simulink model "CusakisME4901delay"  (R2013a)
settings: Solver=ode4  StartTime=0.0  StopTime=inf  FixedStep=0.1  RelTol=1e-3
InitFcn:
  | STEPS=14;
  | STEPVEC=[1 1 1 2 2 2 2 3 3 3 4 4 4 4].';
  | TimeStepAct=0.1;
  | f13=3;%second of second and fourth phase
  | f24=4;%second of second and fourth phase
undefined symbols (not defined in the file or in its folder): serial
libraries: instrumentlib x5, simulink x2, aerolibanimutils x1, vrlib x1
settings Model: Creator=Grompone  LastModifiedBy=Grompone

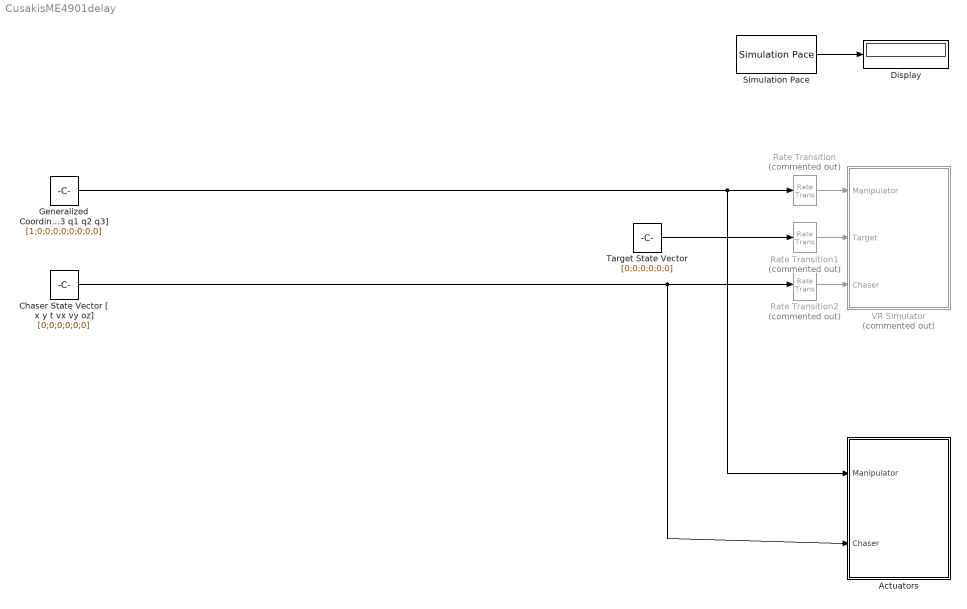
== system CusakisME4901delay ==
  Actuators : Subsystem
  "Chaser State Vector [ x y t vx vy oz] " : Constant  Value=[0;0;0;0;0;0]
  Display : Display
  Generalized Coordinates [qdd1 qdd2 qdd3 qd1 qd2 qd3 q1 q2 q3] : Constant  Value=[1;0;0;0;0;0;0;0;0]
  Rate Transition : RateTransition  Commented=on  OutPortSampleTime=0.2
  Rate Transition1 : RateTransition  Commented=on  OutPortSampleTime=0.2
  Rate Transition2 : RateTransition  Commented=on  OutPortSampleTime=0.2
  Simulation Pace : aerolibanimutils/Simulation Pace  SimulationPace=1  SleepMode=MATLAB Thread  OutputPaceError=on  SampleTime=0.01
      settings: AttributesFormatString=%<SimulationPace> sec/sec
  Target State Vector : Constant  Value=[0;0;0;0;0;0]
  VR Simulator : Subsystem  Commented=on
  wires:
  Rate Transition/1 -> VR Simulator/1(Manipulator)
  Rate Transition1/1 -> VR Simulator/2(Target)
  Rate Transition2/1 -> VR Simulator/3(Chaser)
  Simulation Pace/1 -> Display/1
  "Chaser State Vector [ x y t vx vy oz] "/1 -> Actuators/2(Chaser), Rate Transition2/1
  Target State Vector/1 -> Rate Transition1/1
  Generalized Coordinates [qdd1 qdd2 qdd3 qd1 qd2 qd3 q1 q2 q3]/1 -> Actuators/1(Manipulator), Rate Transition/1

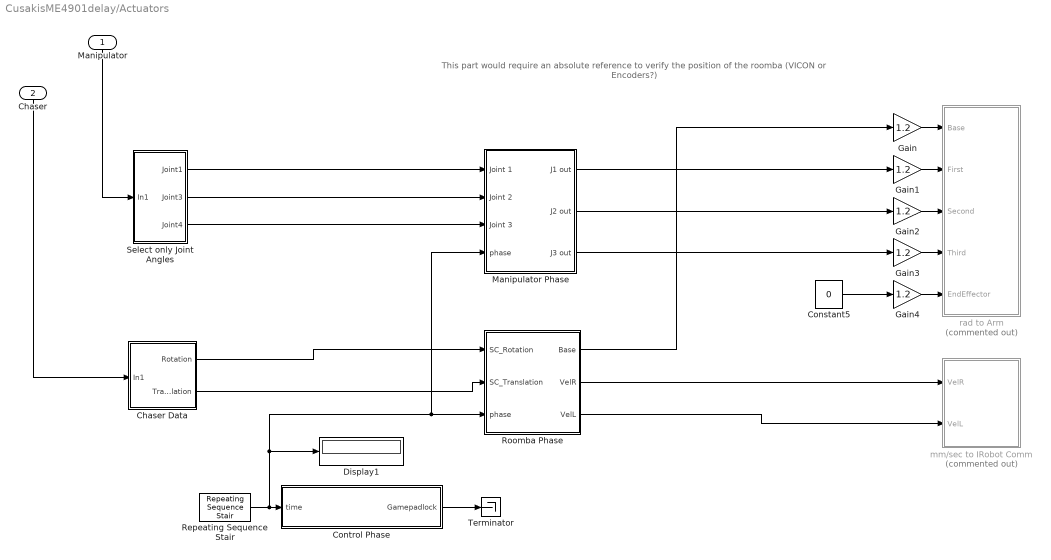
== system CusakisME4901delay/Actuators ==
  note: This part would require an absolute reference to verify the position of the roomba (VICON or Encoders?)
  Manipulator : Inport
  Chaser : Inport  Port=2
  Chaser Data : Subsystem
  Constant5 : Constant  Value=0
  Control Phase : MATLAB Function  TreatAsAtomicUnit=on
  Display1 : Display
  Gain{,1..4} (5 alike) : Gain  Gain=1.2
  Manipulator Phase : Subsystem
  Repeating Sequence Stair : simulink/Sources/Repeating Sequence Stair  OutValues=STEPVEC  tsamp=1  OutMin=[]  OutMax=[]  OutDataTypeStr=double  OutputDataTypeScalingMode=double  OutDataType=fixdt(0,8)  ConRadixGroup=Best Precision: Vector-wise  OutScaling=2^-12
  Roomba Phase : Subsystem
  Select only Joint Angles : Subsystem
  Terminator : Terminator
  mm/sec to IRobot Comm : Subsystem  Commented=on
  rad to Arm : Subsystem  Commented=on
  wires:
  Chaser/1 -> Chaser Data/1(In1)
  Manipulator/1 -> Select only Joint Angles/1(In1)
  Constant5/1 -> Gain4/1
  Chaser Data/2(Translation) -> Roomba Phase/2(SC_Translation)
  Select only Joint Angles/3(Joint4) -> Manipulator Phase/3(Joint 3)
  Select only Joint Angles/2(Joint3) -> Manipulator Phase/2(Joint 2)
  Select only Joint Angles/1(Joint1) -> Manipulator Phase/1(Joint 1)
  Gain/1 -> rad to Arm/1(Base)
  Gain1/1 -> rad to Arm/2(First)
  Gain2/1 -> rad to Arm/3(Second)
  Gain3/1 -> rad to Arm/4(Third)
  Gain4/1 -> rad to Arm/5(EndEffector)
  Chaser Data/1(Rotation) -> Roomba Phase/1(SC_Rotation)
  Manipulator Phase/1(J1 out) -> Gain1/1
  Manipulator Phase/2(J2 out) -> Gain2/1
  Manipulator Phase/3(J3 out) -> Gain3/1
  Repeating Sequence Stair/1 -> Manipulator Phase/4(phase), Roomba Phase/3(phase), Display1/1, Control Phase/1(time)
  Control Phase/1(Gamepadlock) -> Terminator/1
  Roomba Phase/2(VelR) -> mm/sec to IRobot Comm/1(VelR)
  Roomba Phase/3(VelL) -> mm/sec to IRobot Comm/2(VelL)
  Roomba Phase/1(Base) -> Gain/1

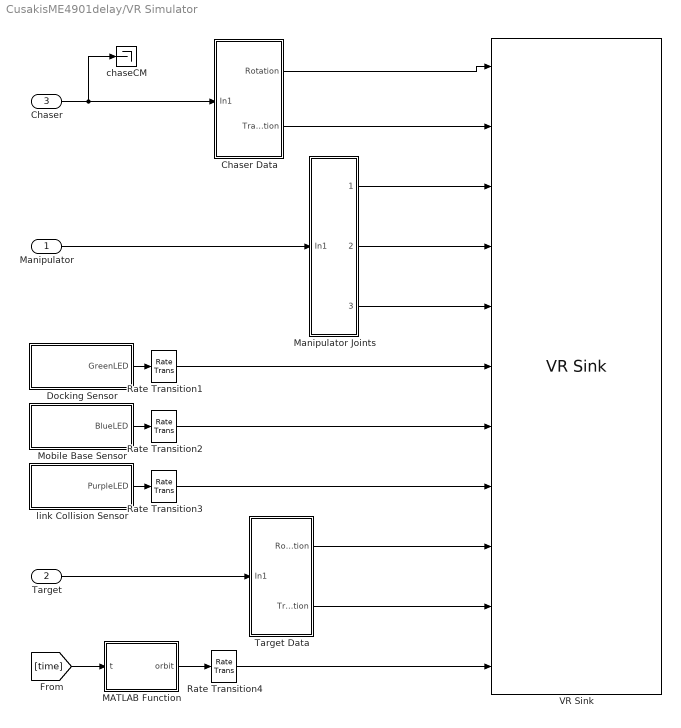
== system CusakisME4901delay/VR Simulator ==
  Manipulator : Inport
  Target : Inport  Port=2
  Chaser : Inport  Port=3
  Chaser Data : Subsystem
  Docking Sensor : Subsystem
  MATLAB Function : MATLAB Function  TreatAsAtomicUnit=on
  Manipulator Joints : Subsystem
  Mobile Base Sensor : Subsystem
  Rate Transition{1..4} (4 alike) : RateTransition  OutPortSampleTime=0.2
  Target Data : Subsystem
  VR Sink : vrlib/VR Sink  InstantiateOnLoad=on  SampleTime=0.2  ViewEnable=on  RemoteChange=off  RemoteView=off  FieldsWritten=CHASER.rotation.4.1.1.double#CHASER.translation.3.1.1.double#Joint1.rotation.4.1.1.double#Joint2.rotation.4.1.1.double#Joint3.rotation.4.1.1.double#we.diffuseColor.3.1.1.double#g.diffuseColor.3.1.1.double#Cl.diffuseColor.3.1.1.double#TARGET.rotation.4.1.1.double#TARGET.translation.3.1.1.double#Otherview.translation.3.1.1.double  WorldFileName=final1b.wrl  AutoView=off  VideoDimensions=[]  AllowVariableSize=off
  chaseCM : Terminator
  link Collision Sensor : Subsystem
  wires:
  Manipulator/1 -> Manipulator Joints/1(In1)
  Target/1 -> Target Data/1(In1)
  [time] -> MATLAB Function/1(t)
  Chaser/1 -> chaseCM/1, Chaser Data/1(In1)
  Chaser Data/1(Rotation) -> VR Sink/1
  Chaser Data/2(Translation) -> VR Sink/2
  Manipulator Joints/1(Joint1) -> VR Sink/3
  Manipulator Joints/3(Joint4) -> VR Sink/5
  Target Data/1(Rotation) -> VR Sink/9
  Target Data/2(Translation) -> VR Sink/10
  MATLAB Function/1(orbit) -> Rate Transition4/1
  link Collision Sensor/1(PurpleLED) -> Rate Transition3/1
  Docking Sensor/1(GreenLED) -> Rate Transition1/1
  Mobile Base Sensor/1(BlueLED) -> Rate Transition2/1
  Manipulator Joints/2(Joint3) -> VR Sink/4
  Rate Transition1/1 -> VR Sink/6
  Rate Transition2/1 -> VR Sink/7
  Rate Transition3/1 -> VR Sink/8
  Rate Transition4/1 -> VR Sink/11

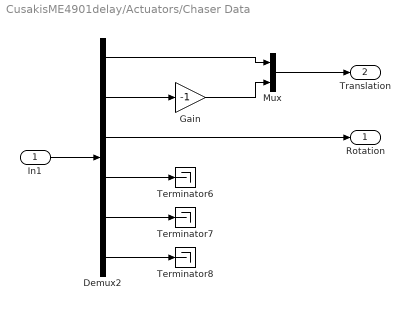
== system CusakisME4901delay/Actuators/Chaser Data ==
  In1 : Inport
  Demux2 : Demux  Outputs=6
  Gain : Gain  Gain=-1
  Mux : Mux  Inputs=2
  Terminator6 : Terminator
  Terminator7 : Terminator
  Terminator8 : Terminator
  Rotation : Outport
  Translation : Outport  Port=2
  wires:
  In1/1 -> Demux2/1
  Demux2/5 -> Terminator7/1
  Demux2/4 -> Terminator6/1
  Demux2/2 -> Gain/1
  Mux/1 -> Translation/1
  Demux2/1 -> Mux/1
  Gain/1 -> Mux/2
  Demux2/3 -> Rotation/1
  Demux2/6 -> Terminator8/1

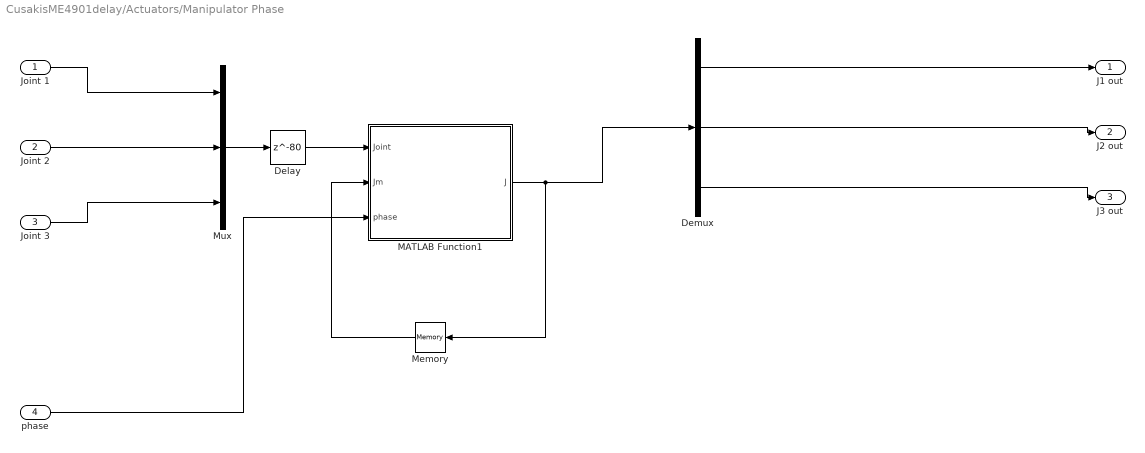
== system CusakisME4901delay/Actuators/Manipulator Phase ==
  Joint 1 : Inport
  Joint 2 : Inport  Port=2
  Joint 3 : Inport  Port=3
  phase : Inport  Port=4
  Delay : Delay  DelayLength=80  InitialCondition=0  SampleTime=0.1
  Demux : Demux  Outputs=3
  MATLAB Function1 : MATLAB Function  TreatAsAtomicUnit=on
  Memory : Memory  X0=[0;0;0]
  Mux : Mux  Inputs=3
  J1 out : Outport
  J2 out : Outport  Port=2
  J3 out : Outport  Port=3
  wires:
  Joint 1/1 -> Mux/1
  Joint 2/1 -> Mux/2
  Joint 3/1 -> Mux/3
  Mux/1 -> Delay/1
  Demux/1 -> J1 out/1
  Demux/2 -> J2 out/1
  Demux/3 -> J3 out/1
  MATLAB Function1/1(J) -> Memory/1, Demux/1
  Memory/1 -> MATLAB Function1/2(Jm)
  phase/1 -> MATLAB Function1/3(phase)
  Delay/1 -> MATLAB Function1/1(Joint)

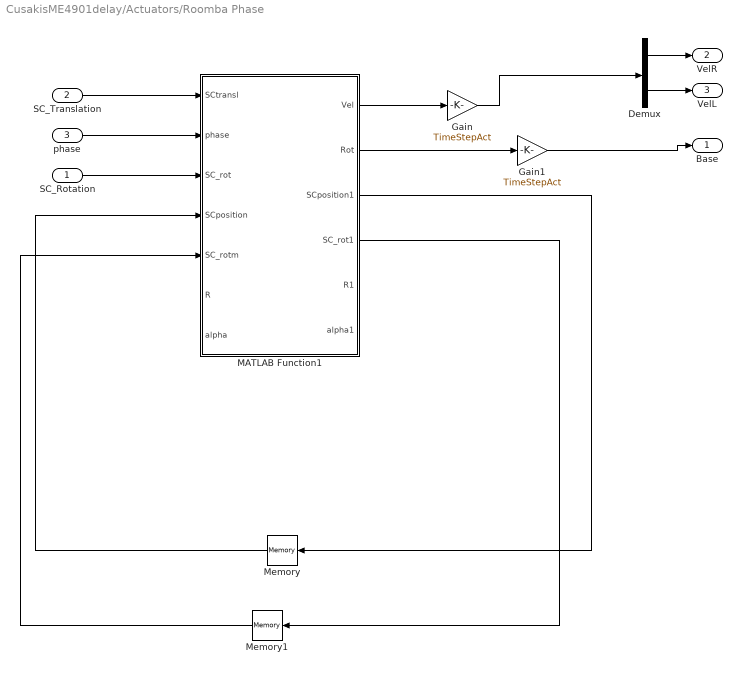
== system CusakisME4901delay/Actuators/Roomba Phase ==
  SC_Rotation : Inport
  SC_Translation : Inport  Port=2
  phase : Inport  Port=3
  Demux : Demux  Outputs=2
  Gain : Gain  Gain=TimeStepAct
  Gain1 : Gain  Gain=TimeStepAct
  MATLAB Function1 : MATLAB Function  TreatAsAtomicUnit=on
  Memory : Memory  X0=[0;0;0]
  Memory1 : Memory
  Base : Outport
  VelR : Outport  Port=2
  VelL : Outport  Port=3
  wires:
  Demux/1 -> VelR/1
  Demux/2 -> VelL/1
  SC_Rotation/1 -> MATLAB Function1/3(SC_rot)
  phase/1 -> MATLAB Function1/2(phase)
  SC_Translation/1 -> MATLAB Function1/1(SCtransl)
  Memory/1 -> MATLAB Function1/4(SCposition)
  Memory1/1 -> MATLAB Function1/5(SC_rotm)
  MATLAB Function1/1(Vel) -> Gain/1
  MATLAB Function1/2(Rot) -> Gain1/1
  MATLAB Function1/3(SCposition1) -> Memory/1
  MATLAB Function1/4(SC_rot1) -> Memory1/1
  Gain/1 -> Demux/1
  Gain1/1 -> Base/1

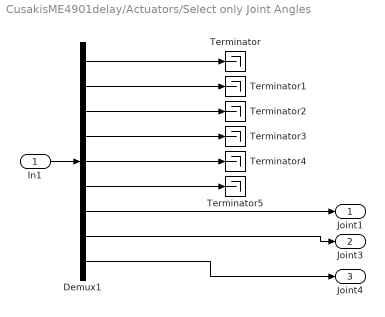
== system CusakisME4901delay/Actuators/Select only Joint Angles ==
  In1 : Inport
  Demux1 : Demux  Outputs=9
  Terminator{,1..5} (6 alike) : Terminator
  Joint1 : Outport
  Joint3 : Outport  Port=2
  Joint4 : Outport  Port=3
  wires:
  Demux1/9 -> Joint4/1
  Demux1/8 -> Joint3/1
  Demux1/7 -> Joint1/1
  Demux1/6 -> Terminator5/1
  Demux1/5 -> Terminator4/1
  Demux1/4 -> Terminator3/1
  Demux1/3 -> Terminator2/1
  Demux1/2 -> Terminator1/1
  Demux1/1 -> Terminator/1
  In1/1 -> Demux1/1

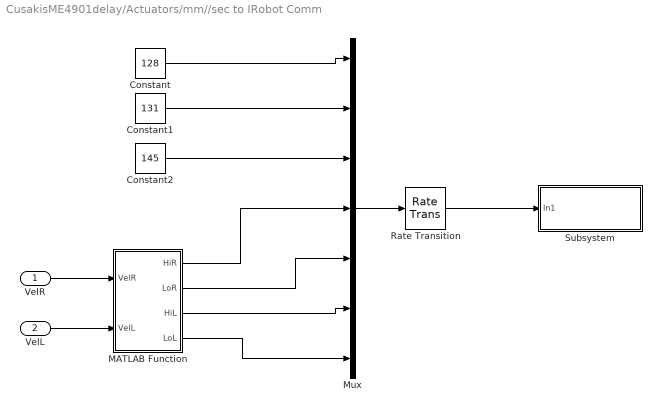
== system CusakisME4901delay/Actuators/mm//sec to IRobot Comm ==
  VelR : Inport
  VelL : Inport  Port=2
  Constant : Constant  Value=128  OutDataTypeStr=uint8
  Constant1 : Constant  Value=131  OutDataTypeStr=uint8
  Constant2 : Constant  Value=145  OutDataTypeStr=uint8
  MATLAB Function : MATLAB Function  TreatAsAtomicUnit=on
  Mux : Mux  Inputs=7
  Rate Transition : RateTransition  OutPortSampleTime=1
  Subsystem : Subsystem
  wires:
  MATLAB Function/1(HiR) -> Mux/4
  MATLAB Function/2(LoR) -> Mux/5
  MATLAB Function/3(HiL) -> Mux/6
  MATLAB Function/4(LoL) -> Mux/7
  VelR/1 -> MATLAB Function/1(VelR)
  VelL/1 -> MATLAB Function/2(VelL)
  Constant/1 -> Mux/1
  Constant1/1 -> Mux/2
  Constant2/1 -> Mux/3
  Mux/1 -> Rate Transition/1
  Rate Transition/1 -> Subsystem/1(In1)

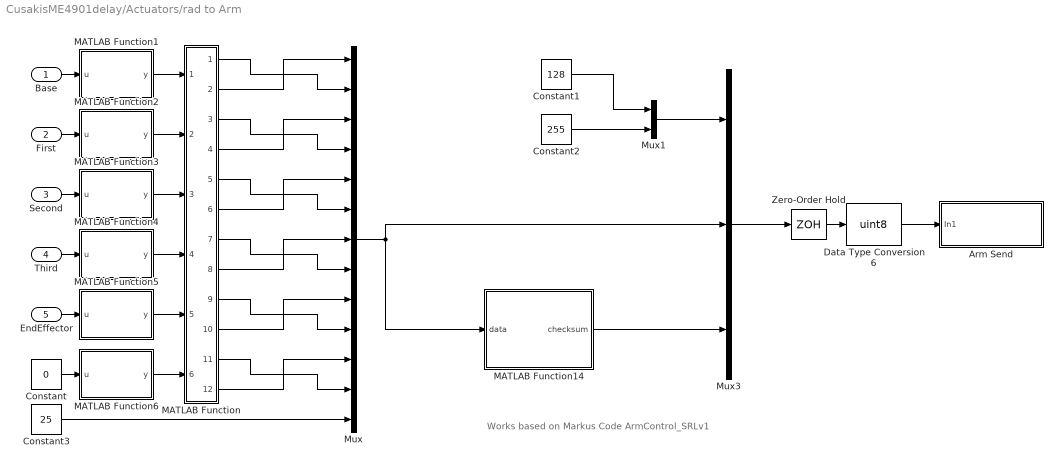
== system CusakisME4901delay/Actuators/rad to Arm ==
  note: Works based on Markus Code ArmControl_SRLv1
  Base : Inport
  First : Inport  Port=2
  Second : Inport  Port=3
  Third : Inport  Port=4
  EndEffector : Inport  Port=5
  Arm Send : Subsystem
  Constant : Constant  Value=0  OutDataTypeStr=uint8
  Constant1 : Constant  Value=128  OutDataTypeStr=uint8
  Constant2 : Constant  Value=255  OutDataTypeStr=uint8
  Constant3 : Constant  Value=25  OutDataTypeStr=uint8
  Data Type Conversion6 : DataTypeConversion  OutDataTypeStr=uint8
  MATLAB Function : MATLAB Function  TreatAsAtomicUnit=on
  MATLAB Function1 : MATLAB Function  TreatAsAtomicUnit=on
  MATLAB Function14 : MATLAB Function  TreatAsAtomicUnit=on
  MATLAB Function2 : MATLAB Function  TreatAsAtomicUnit=on
  MATLAB Function3 : MATLAB Function  TreatAsAtomicUnit=on
  MATLAB Function4 : MATLAB Function  TreatAsAtomicUnit=on
  MATLAB Function5 : MATLAB Function  TreatAsAtomicUnit=on
  MATLAB Function6 : MATLAB Function  TreatAsAtomicUnit=on
  Mux : Mux  Inputs=13
  Mux1 : Mux  Inputs=2
  Mux3 : Mux  Inputs=3
  Zero-Order Hold : ZeroOrderHold  SampleTime=0.01
  wires:
  EndEffector/1 -> MATLAB Function5/1(u)
  First/1 -> MATLAB Function2/1(u)
  Second/1 -> MATLAB Function3/1(u)
  Third/1 -> MATLAB Function4/1(u)
  Base/1 -> MATLAB Function1/1(u)
  Constant/1 -> MATLAB Function6/1(u)
  Constant1/1 -> Mux1/1
  Constant2/1 -> Mux1/2
  Constant3/1 -> Mux/13
  MATLAB Function14/1(checksum) -> Mux3/3
  Mux/1 -> Mux3/2, MATLAB Function14/1(data)
  Mux1/1 -> Mux3/1
  Data Type Conversion6/1 -> Arm Send/1(In1)
  MATLAB Function/2(LoBase) -> Mux/1
  MATLAB Function/4(LoM1) -> Mux/3
  MATLAB Function/6(LoM2) -> Mux/5
  MATLAB Function/8(LoM3) -> Mux/7
  MATLAB Function/10(LoEnd) -> Mux/9
  MATLAB Function/12(LoO) -> Mux/11
  MATLAB Function/1(HiBase) -> Mux/2
  MATLAB Function/3(HiM1) -> Mux/4
  MATLAB Function/5(HiM2) -> Mux/6
  MATLAB Function/7(HiM3) -> Mux/8
  MATLAB Function/9(HiEnd) -> Mux/10
  MATLAB Function/11(HiO) -> Mux/12
  MATLAB Function1/1(y) -> MATLAB Function/1(Base)
  MATLAB Function2/1(y) -> MATLAB Function/2(M1)
  MATLAB Function3/1(y) -> MATLAB Function/3(M2)
  MATLAB Function4/1(y) -> MATLAB Function/4(M3)
  MATLAB Function5/1(y) -> MATLAB Function/5(End)
  MATLAB Function6/1(y) -> MATLAB Function/6(other)
  Mux3/1 -> Zero-Order Hold/1
  Zero-Order Hold/1 -> Data Type Conversion6/1

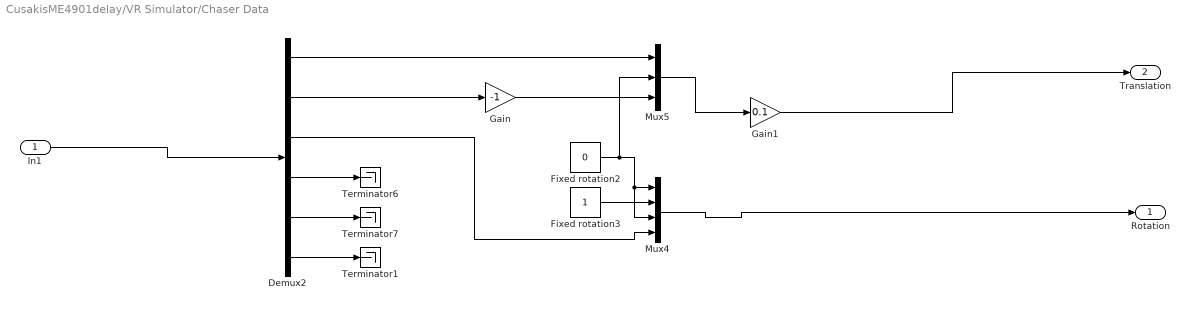
== system CusakisME4901delay/VR Simulator/Chaser Data ==
  In1 : Inport
  Demux2 : Demux  Outputs=6
  Fixed rotation2 : Constant  Value=0
  Fixed rotation3 : Constant
  Gain : Gain  Gain=-1
  Gain1 : Gain  Gain=0.1
  Mux4 : Mux
  Mux5 : Mux  Inputs=3
  Terminator1 : Terminator
  Terminator6 : Terminator
  Terminator7 : Terminator
  Rotation : Outport
  Translation : Outport  Port=2
  wires:
  In1/1 -> Demux2/1
  Mux5/1 -> Gain1/1
  Demux2/5 -> Terminator7/1
  Demux2/4 -> Terminator6/1
  Demux2/2 -> Gain/1
  Fixed rotation2/1 -> Mux4/1, Mux4/3, Mux5/2
  Fixed rotation3/1 -> Mux4/2
  Demux2/3 -> Mux4/4
  Gain1/1 -> Translation/1
  Mux4/1 -> Rotation/1
  Demux2/1 -> Mux5/1
  Gain/1 -> Mux5/3
  Demux2/6 -> Terminator1/1

== system CusakisME4901delay/VR Simulator/Docking Sensor ==
  Fixed translation3 : Constant  Value=[0 0 0]
  Green : Constant  Value=[0.2 1 0.2]
  Rate Transition : RateTransition
  Red : Constant  Value=[1 0 0]
  Repeating Sequence Stair : simulink/Sources/Repeating Sequence Stair  OutValues=[0 1].'  tsamp=0.5  OutMin=[]  OutMax=[]  OutDataTypeStr=double  OutputDataTypeScalingMode=double  OutDataType=fixdt(0,8)  ConRadixGroup=Best Precision: Vector-wise  OutScaling=2^-12
  Switch : Switch  Criteria=u2 ~= 0
  Switch1 : Switch  Criteria=u2 ~= 0
  GreenLED : Outport
  wires:
  [docking] -> Switch/2
  Fixed translation3/1 -> Switch1/3
  Repeating Sequence Stair/1 -> Rate Transition/1
  Green/1 -> Switch/1
  Red/1 -> Switch1/1
  Switch1/1 -> Switch/3
  Rate Transition/1 -> Switch1/2
  Switch/1 -> GreenLED/1

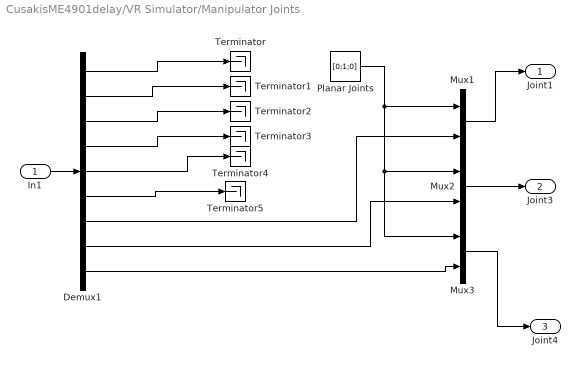
== system CusakisME4901delay/VR Simulator/Manipulator Joints ==
  In1 : Inport
  Demux1 : Demux  Outputs=9
  Mux1 : Mux  Inputs=2
  Mux2 : Mux  Inputs=2
  Mux3 : Mux  Inputs=2
  Planar Joints : Constant  Value=[0;1;0]
  Terminator{,1..5} (6 alike) : Terminator
  Joint1 : Outport
  Joint3 : Outport  Port=2
  Joint4 : Outport  Port=3
  wires:
  In1/1 -> Demux1/1
  Demux1/8 -> Mux2/2
  Demux1/9 -> Mux3/2
  Demux1/7 -> Mux1/2
  Demux1/1 -> Terminator/1
  Demux1/2 -> Terminator1/1
  Demux1/3 -> Terminator2/1
  Demux1/4 -> Terminator3/1
  Demux1/5 -> Terminator4/1
  Demux1/6 -> Terminator5/1
  Planar Joints/1 -> Mux3/1, Mux2/1, Mux1/1
  Mux1/1 -> Joint1/1
  Mux2/1 -> Joint3/1
  Mux3/1 -> Joint4/1

== system CusakisME4901delay/VR Simulator/Mobile Base Sensor ==
  Green : Constant  Value=[0 0 0]
  Green1 : Constant  Value=[0 0 1]
  Switch : Switch  Criteria=u2 ~= 0
  BlueLED : Outport
  wires:
  Switch/1 -> BlueLED/1
  Green/1 -> Switch/1
  [mobilebase] -> Switch/2
  Green1/1 -> Switch/3

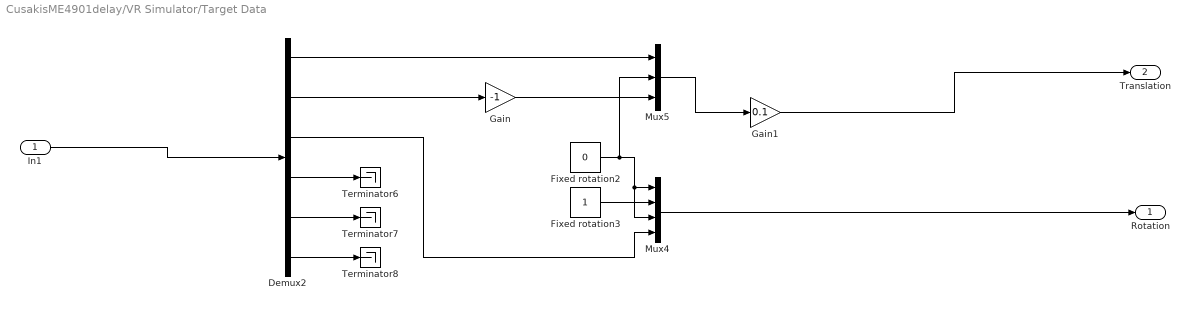
== system CusakisME4901delay/VR Simulator/Target Data ==
  In1 : Inport
  Demux2 : Demux  Outputs=6
  Fixed rotation2 : Constant  Value=0
  Fixed rotation3 : Constant
  Gain : Gain  Gain=-1
  Gain1 : Gain  Gain=0.1
  Mux4 : Mux
  Mux5 : Mux  Inputs=3
  Terminator6 : Terminator
  Terminator7 : Terminator
  Terminator8 : Terminator
  Rotation : Outport
  Translation : Outport  Port=2
  wires:
  Fixed rotation3/1 -> Mux4/2
  Fixed rotation2/1 -> Mux5/2, Mux4/3, Mux4/1
  Demux2/1 -> Mux5/1
  Demux2/2 -> Gain/1
  Demux2/3 -> Mux4/4
  Demux2/4 -> Terminator6/1
  Demux2/5 -> Terminator7/1
  Demux2/6 -> Terminator8/1
  Gain/1 -> Mux5/3
  Mux5/1 -> Gain1/1
  Gain1/1 -> Translation/1
  Mux4/1 -> Rotation/1
  In1/1 -> Demux2/1

== system CusakisME4901delay/VR Simulator/link Collision Sensor ==
  Black : Constant  Value=[0 0 0]
  Purple : Constant  Value=[1 0 1]
  Switch : Switch  Criteria=u2 ~= 0
  PurpleLED : Outport
  wires:
  Black/1 -> Switch/3
  [linkcoll] -> Switch/2
  Purple/1 -> Switch/1
  Switch/1 -> PurpleLED/1

== system CusakisME4901delay/Actuators/mm//sec to IRobot Comm/Subsystem ==
  In1 : Inport
  Serial Configuration : instrumentlib/Serial Configuration  Priority=-200000  ComPortMenu=<Please select a port...>  ComPort=COM4  ObjConstructor=serial('COM4');  BaudRate=57600  DataBits=8  Parity=none  StopBits=1  FlowControl=none  Timeout=10  ByteOrder=LittleEndian
  Serial Send : instrumentlib/Serial Send  ComPortMenu=<Please select a port...>  ComPort=COM4  ObjConstructor=serial('COM4');  Terminator=<none>  EnableBlockingMode=off
  wires:
  In1/1 -> Serial Send/1

== system CusakisME4901delay/Actuators/rad to Arm/Arm Send ==
  In1 : Inport
  Display2 : Display
  Display3 : Display
  Rate Transition : RateTransition  OutPortSampleTime=0.1
  Serial Configuration : instrumentlib/Serial Configuration  Priority=-200000  ComPortMenu=<Please select a port...>  ComPort=COM5  ObjConstructor=serial('COM5');  BaudRate=57600  DataBits=8  Parity=none  StopBits=1  FlowControl=none  Timeout=10  ByteOrder=LittleEndian
  Serial Receive : instrumentlib/Serial Receive  ComPortMenu=<Please select a port...>  ComPort=COM5  ObjConstructor=serial('COM5');  Terminator=<none>  DataSize="[1  16]"  DataType=uint8  EnableBlockingMode=off  ActionDataUnavailable=Output last received value  CustomValue=0  SampleTime=0.1
  Serial Send : instrumentlib/Serial Send  ComPortMenu=<Please select a port...>  ComPort=COM5  ObjConstructor=serial('COM5');  Terminator=<none>  EnableBlockingMode=off
  wires:
  In1/1 -> Rate Transition/1
  Rate Transition/1 -> Serial Send/1
  Serial Receive/1 -> Display2/1
  Serial Receive/2 -> Display3/1

== matlab function CusakisME4901delay/Actuators/Roomba Phase/MATLAB Function1 ==
  data: SCtransl input; phase input; SC_rot input; SCposition input; Vel output; SC_rotm input; R input; alpha input; Rot output; f13 parameter; f24 parameter; SCposition1 output; SC_rot1 output; R1 output; alpha1 output
function [Vel,Rot,SCposition1,SC_rot1,R1,alpha1]  = fcn(SCtransl,phase,SC_rot,SCposition,SC_rotm,R,alpha,f13,f24)
%#codegen

%Inputs
r=0.13; %radius of roomba's wheels
%SCtranslation [ X; Y; Theta; Vx; Vy; Omega ]

%SCposition [X; Y; Theta]

if phase==1 %CONTROL PHASE Operator is giving the inputs and the time history is being computed
    SCposition1=SCposition;
    SC_rot1=SC_rot;
    
    Vel=[0;0];
    Rot=SC_rotm;

elseif phase==2 %ADAPTATION PHASE The base adapts it's attitude in order to be ready to maneuver and the velocities are 0
    SCposition1=SCposition;
    SC_rot1=SC_rot;
    
    Xf=SCposition;
    Xi=SCtransl;
    DeltaSC=[Xf(1)-Xi(1);Xf(2)-Xi(2);Xf(3)-Xi(3)];
    
    R=sqrt(DelataSC(1)^2+DelataSC(2)^2); %distance to maneuvered
    
    alpha=atan2(DeltaSC(2),DeltaSC(1));  %angle to be maneuvered
    
    if alpha>0 && alpha <1.57
        Sl=alpha*(-r);
        Sr=alpha*(r);
    elseif alpha>1.57 && alpha <3.14
        Sl=alpha*(-r);
        Sr=alpha*(r);
    elseif alpha<0 && alpha >-1.57
        Sl=-alpha*(r);
        Sr=-alpha*(-r);
    elseif alpha<-1.57 && alpha >-3.14
        Sl=-alpha*(r);
        Sr=-alpha*(-r);
    end
    
    %this part should be integrated....in steps to regulate velocity!!
    Vel=[Sr/f24;Sl/f24]; %Provides only the angle maneuver
    Rot=-alpha/f24; %the First Link has to compensate this adaptation
     
elseif phase==3 %SIMULATION PHASE Manipulator and base maneuver according to time history
    SCposition1=SCposition;
    SC_rot1=SC_rot;
    
    %Simulates translation of the spacecraft time histories
    Vel=[R/f13;R/f13];
    Rot=SC_rot; %simulates rotations of the spacecraft time histories
    
else %RESET PHASE, Cancels angle between base and Roomba
    SCposition1=SCtransl;
    SC_rot1=SC_rotm;
    
    Rot=SC_rot+Rot; %simulates rotations of the spacecraft time histories
    Vel=[R/f13;R/f13];
    
end

== matlab function CusakisME4901delay/Actuators/Control Phase ==
  data: time input; Gamepadlock output
function Gamepadlock = fcn(time)
%#codegen



if time==1 
    
Gamepadlock=1; 

else
    
Gamepadlock=0;  %Locks the gamepad when the user cannot send data.  

end


%What I Want from this code


% if time<3*n
%     
% Joypad inputs the velocities and the model calculates the generalized
% coordinates and spacecraft position
%
%
% if time>3*n && time<8*n
%
% The model stops computation saves the time history of the gen coordinates
% The Cusakis rotates towards the direction it will have to move
%
%
% if time>8*n && time<11*n
%
% Cusakis moves twoards the new center position and the manipulator uses
% the time history 
%
%

== matlab function CusakisME4901delay/Actuators/Manipulator Phase/MATLAB Function1 ==
  data: Joint input; Jm input; phase input; J output
function J   = fcn(Joint,Jm,phase)
%#codegen

%freeses the manipulator in phase 1 2 and 4


if phase==3 
      J=Joint;
else
    J=Jm;
end

== matlab function CusakisME4901delay/VR Simulator/MATLAB Function ==
  data: t input; orbit output
function orbit = fcn(t)
%#codegen



w=0.01;

x=cos(w*t);

z=sin(w*t);

y=0;

%orbit = [x;y;z];

orbit = [0;0;0];

== matlab function CusakisME4901delay/Actuators/rad to Arm/MATLAB Function1 ==
  data: u input; y output
function y = fcn(u)
%#codegen
udeg=u*180/pi;

%degrees to arduino angles..(avoids negative numbers)
y = (udeg+180)*10;

== matlab function CusakisME4901delay/Actuators/rad to Arm/MATLAB Function2 ==
  data: u input; y output
function y = fcn(u)
%#codegen
udeg=u*180/pi;

%degrees to arduino angles..(avoids negative numbers)
y = (udeg+180)*10;

== matlab function CusakisME4901delay/Actuators/rad to Arm/MATLAB Function3 ==
  data: u input; y output
function y = fcn(u)
%#codegen
udeg=u*180/pi;

%degrees to arduino angles..(avoids negative numbers)
y = (udeg+180)*10;

== matlab function CusakisME4901delay/Actuators/rad to Arm/MATLAB Function4 ==
  data: u input; y output
function y = fcn(u)
%#codegen
udeg=u*180/pi;

%degrees to arduino angles..(avoids negative numbers)
y = (udeg+180)*10;

== matlab function CusakisME4901delay/Actuators/rad to Arm/MATLAB Function5 ==
  data: u input; y output
function y = fcn(u)
%#codegen
udeg=u*180/pi;

%degrees to arduino angles..(avoids negative numbers)
y = (udeg+180)*10;

== matlab function CusakisME4901delay/Actuators/rad to Arm/MATLAB Function ==
  data: Base input; HiBase output; M1 input; LoBase output; HiM1 output; LoM1 output; M2 input; M3 input; End input; HiM2 output; LoM2 output; HiM3 output; LoM3 output; HiEnd output; LoEnd output; other input; HiO output; LoO output
function [HiBase,LoBase,HiM1,LoM1,HiM2,LoM2,HiM3,LoM3,HiEnd,LoEnd,HiO,LoO] = fcn(Base,M1,M2,M3,End,other)
%#codegen


BaseV=typecast(int16(Base),'uint8');
M1V=typecast(int16(M1),'uint8');
M2V=typecast(int16(M2),'uint8');
M3V=typecast(int16(M3),'uint8');
EndV=typecast(int16(End),'uint8');
OtherV=typecast(int16(other),'uint8');


HiBase=BaseV(2);
LoBase=BaseV(1);
HiM1=M1V(2);
LoM1=M1V(1);
HiM2=M2V(2);
LoM2=M2V(1);
HiM3=M3V(2);
LoM3=M3V(1);
HiEnd=EndV(2);
LoEnd=EndV(1);
HiO=OtherV(2);
LoO=OtherV(1);

== matlab function CusakisME4901delay/Actuators/rad to Arm/MATLAB Function14 ==
  data: data input; checksum output
function checksum = Checksum(data)
% Calculates checksum of command signal

data = int16(data);
tempsum = sum(data);
temp = 255 - mod(tempsum,256);

checksum = uint8(temp);

== matlab function CusakisME4901delay/Actuators/rad to Arm/MATLAB Function6 ==
  data: u input; y output
function y = fcn(u)
%#codegen
udeg=u*180/pi;

%degrees to arduino angles..(avoids negative numbers)
y = (udeg+180)*10;

== matlab function CusakisME4901delay/Actuators/mm//sec to IRobot Comm/MATLAB Function ==
  data: VelR input; HiR output; VelL input; LoR output; HiL output; LoL output
function [HiR,LoR,HiL,LoL] = fcn(VelR,VelL)
%#codegen


%max velocity 500 mm/s 0.5 m/s


R=typecast(int16(VelR),'uint8');
 %typecast(int16(-200),'uint8')
 
HiR=R(2);
LoR=R(1);

L=typecast(int16(VelL),'uint8');
 %typecast(int16(-200),'uint8')
 
HiL=L(2);
LoL=L(1);
